simulink model "FPU_integrator"  (Simulink 7.6)
settings: Solver=FixedStepDiscrete  StartTime=0.0  StopTime=50  FixedStep=1  RelTol=1e-3
libraries: simulink x6
settings Model: Creator=jordan  LastModifiedBy=jordan
settings OptimizationCC: BlockReduction=off  ConditionallyExecuteInputs=off

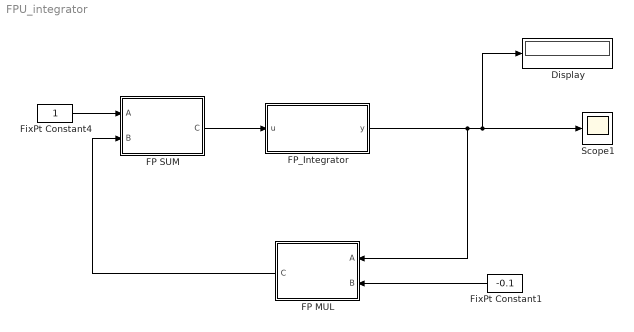
== system FPU_integrator ==
  Display : Display
  FP MUL : Subsystem
  FP SUM : Subsystem
  FP_Integrator : Subsystem
  FixPt Constant1 : Constant  DisableCoverage=on  Value=-0.1  OutDataTypeStr=single  LockScale=on
  FixPt Constant4 : Constant  DisableCoverage=on  OutDataTypeStr=single  LockScale=on
  Scope1 : Scope
      settings: SaveName=ScopeData3  MaxDataPoints=50000
  wires:
  FP_Integrator/1(y) -> Scope1/1, Display/1, FP MUL/1(A)
  FixPt Constant4/1 -> FP SUM/1(A)
  FixPt Constant1/1 -> FP MUL/2(B)
  FP SUM/1(C) -> FP_Integrator/1(u)
  FP MUL/1(C) -> FP SUM/2(B)

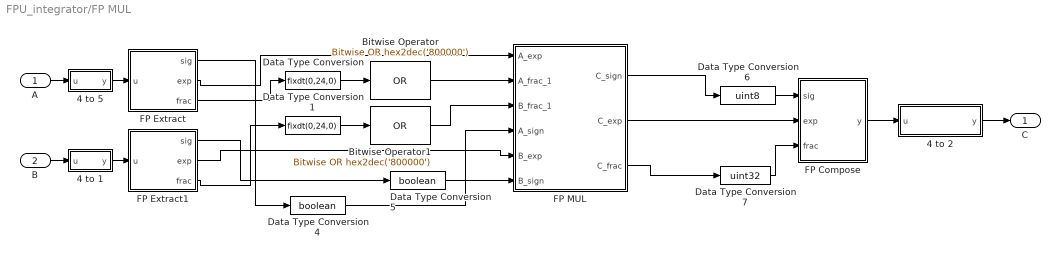
== system FPU_integrator/FP MUL ==
  A : Inport
  B : Inport  Port=2
  4 to 1 : Stateflow chart  TreatAsAtomicUnit=on
  4 to 2 : Stateflow chart  TreatAsAtomicUnit=on
  4 to 5 : Stateflow chart  TreatAsAtomicUnit=on
  Bitwise Operator : simulink/Logic and Bit Operations/Bitwise Operator  logicop=OR  UseBitMask=on  BitMask=hex2dec('800000')  BitMaskRealWorld=Stored Integer
  Bitwise Operator1 : simulink/Logic and Bit Operations/Bitwise Operator  logicop=OR  UseBitMask=on  BitMask=hex2dec('800000')  BitMaskRealWorld=Stored Integer
  Data Type Conversion : DataTypeConversion  OutDataTypeStr=fixdt(0,24,0)  RndMeth=Nearest
  Data Type Conversion1 : DataTypeConversion  OutDataTypeStr=fixdt(0,24,0)  RndMeth=Nearest
  Data Type Conversion4 : DataTypeConversion  OutDataTypeStr=boolean  RndMeth=Nearest
  Data Type Conversion5 : DataTypeConversion  OutDataTypeStr=boolean  RndMeth=Nearest
  Data Type Conversion6 : DataTypeConversion  OutDataTypeStr=uint8  RndMeth=Nearest
  Data Type Conversion7 : DataTypeConversion  OutDataTypeStr=uint32  RndMeth=Nearest
  FP Compose : Stateflow chart  TreatAsAtomicUnit=on
  FP Extract : Stateflow chart  TreatAsAtomicUnit=on
  FP Extract1 : Stateflow chart  TreatAsAtomicUnit=on
  FP MUL : Subsystem
  C : Outport  InitialOutput=0
  wires:
  Data Type Conversion7/1 -> FP Compose/3(frac)
  Data Type Conversion6/1 -> FP Compose/1(sig)
  FP Compose/1(y) -> 4 to 2/1(u)
  Data Type Conversion5/1 -> FP MUL/6(B_sign)
  Data Type Conversion4/1 -> FP MUL/4(A_sign)
  FP MUL/3(C_frac) -> Data Type Conversion7/1
  FP MUL/2(C_exp) -> FP Compose/2(exp)
  FP MUL/1(C_sign) -> Data Type Conversion6/1
  Bitwise Operator1/1 -> FP MUL/3(B_frac_1)
  Data Type Conversion1/1 -> Bitwise Operator1/1
  Bitwise Operator/1 -> FP MUL/2(A_frac_1)
  Data Type Conversion/1 -> Bitwise Operator/1
  FP Extract1/3(frac) -> Data Type Conversion1/1
  FP Extract/3(frac) -> Data Type Conversion/1
  FP Extract1/2(exp) -> FP MUL/5(B_exp)
  FP Extract/2(exp) -> FP MUL/1(A_exp)
  FP Extract1/1(sig) -> Data Type Conversion5/1
  FP Extract/1(sig) -> Data Type Conversion4/1
  B/1 -> 4 to 1/1(u)
  A/1 -> 4 to 5/1(u)
  4 to 5/1(y) -> FP Extract/1(u)
  4 to 1/1(y) -> FP Extract1/1(u)
  4 to 2/1(y) -> C/1

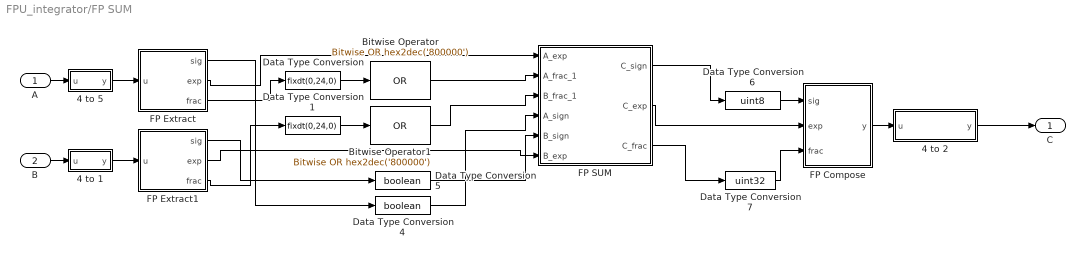
== system FPU_integrator/FP SUM ==
  A : Inport
  B : Inport  Port=2
  4 to 1 : Stateflow chart  TreatAsAtomicUnit=on
  4 to 2 : Stateflow chart  TreatAsAtomicUnit=on
  4 to 5 : Stateflow chart  TreatAsAtomicUnit=on
  Bitwise Operator : simulink/Logic and Bit Operations/Bitwise Operator  logicop=OR  UseBitMask=on  BitMask=hex2dec('800000')  BitMaskRealWorld=Stored Integer
  Bitwise Operator1 : simulink/Logic and Bit Operations/Bitwise Operator  logicop=OR  UseBitMask=on  BitMask=hex2dec('800000')  BitMaskRealWorld=Stored Integer
  Data Type Conversion : DataTypeConversion  OutDataTypeStr=fixdt(0,24,0)  RndMeth=Nearest
  Data Type Conversion1 : DataTypeConversion  OutDataTypeStr=fixdt(0,24,0)  RndMeth=Nearest
  Data Type Conversion4 : DataTypeConversion  OutDataTypeStr=boolean  RndMeth=Nearest
  Data Type Conversion5 : DataTypeConversion  OutDataTypeStr=boolean  RndMeth=Nearest
  Data Type Conversion6 : DataTypeConversion  OutDataTypeStr=uint8  RndMeth=Nearest
  Data Type Conversion7 : DataTypeConversion  OutDataTypeStr=uint32  RndMeth=Nearest
  FP Compose : Stateflow chart  TreatAsAtomicUnit=on
  FP Extract : Stateflow chart  TreatAsAtomicUnit=on
  FP Extract1 : Stateflow chart  TreatAsAtomicUnit=on
  FP SUM : Subsystem
  C : Outport  InitialOutput=0
  wires:
  A/1 -> 4 to 5/1(u)
  B/1 -> 4 to 1/1(u)
  FP Extract/1(sig) -> Data Type Conversion4/1
  FP Extract1/1(sig) -> Data Type Conversion5/1
  FP Extract/2(exp) -> FP SUM/1(A_exp)
  FP Extract1/2(exp) -> FP SUM/6(B_exp)
  FP Extract/3(frac) -> Data Type Conversion/1
  FP Extract1/3(frac) -> Data Type Conversion1/1
  Data Type Conversion/1 -> Bitwise Operator/1
  Bitwise Operator/1 -> FP SUM/2(A_frac_1)
  Data Type Conversion1/1 -> Bitwise Operator1/1
  Bitwise Operator1/1 -> FP SUM/3(B_frac_1)
  FP SUM/1(C_sign) -> Data Type Conversion6/1
  FP SUM/2(C_exp) -> FP Compose/2(exp)
  FP SUM/3(C_frac) -> Data Type Conversion7/1
  Data Type Conversion4/1 -> FP SUM/4(A_sign)
  Data Type Conversion5/1 -> FP SUM/5(B_sign)
  FP Compose/1(y) -> 4 to 2/1(u)
  Data Type Conversion6/1 -> FP Compose/1(sig)
  Data Type Conversion7/1 -> FP Compose/3(frac)
  4 to 5/1(y) -> FP Extract/1(u)
  4 to 1/1(y) -> FP Extract1/1(u)
  4 to 2/1(y) -> C/1

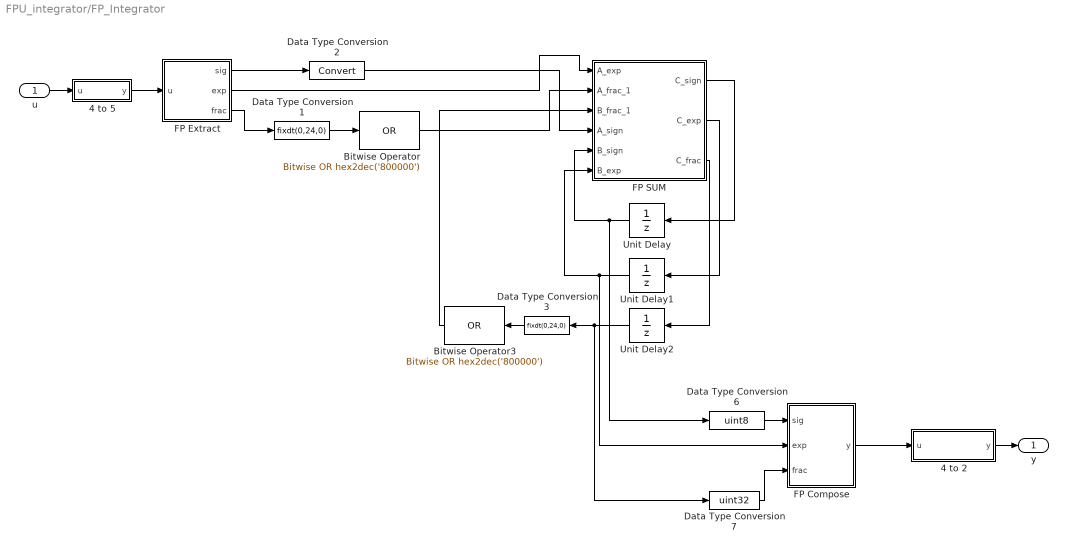
== system FPU_integrator/FP_Integrator ==
  u : Inport
  4 to 2 : Stateflow chart  TreatAsAtomicUnit=on
  4 to 5 : Stateflow chart  TreatAsAtomicUnit=on
  Bitwise Operator : simulink/Logic and Bit Operations/Bitwise Operator  logicop=OR  UseBitMask=on  BitMask=hex2dec('800000')  BitMaskRealWorld=Stored Integer
  Bitwise Operator3 : simulink/Logic and Bit Operations/Bitwise Operator  logicop=OR  UseBitMask=on  BitMask=hex2dec('800000')  BitMaskRealWorld=Stored Integer
  Data Type Conversion1 : DataTypeConversion  OutDataTypeStr=fixdt(0,24,0)  RndMeth=Nearest
  Data Type Conversion2 : DataTypeConversion  RndMeth=Nearest
  Data Type Conversion3 : DataTypeConversion  OutDataTypeStr=fixdt(0,24,0)  RndMeth=Nearest
  Data Type Conversion6 : DataTypeConversion  OutDataTypeStr=uint8  RndMeth=Nearest
  Data Type Conversion7 : DataTypeConversion  OutDataTypeStr=uint32  RndMeth=Nearest
  FP Compose : Stateflow chart  TreatAsAtomicUnit=on
  FP Extract : Stateflow chart  TreatAsAtomicUnit=on
  FP SUM : Subsystem
  Unit Delay : UnitDelay  SampleTime=-1
  Unit Delay1 : UnitDelay  SampleTime=-1
  Unit Delay2 : UnitDelay  SampleTime=-1
  y : Outport
  wires:
  FP SUM/1(C_sign) -> Unit Delay/1
  FP SUM/2(C_exp) -> Unit Delay1/1
  FP SUM/3(C_frac) -> Unit Delay2/1
  Unit Delay/1 -> FP SUM/5(B_sign), Data Type Conversion6/1
  Unit Delay1/1 -> FP SUM/6(B_exp), FP Compose/2(exp)
  Unit Delay2/1 -> Data Type Conversion3/1, Data Type Conversion7/1
  Data Type Conversion3/1 -> Bitwise Operator3/1
  Bitwise Operator3/1 -> FP SUM/3(B_frac_1)
  FP Extract/1(sig) -> Data Type Conversion2/1
  FP Extract/2(exp) -> FP SUM/1(A_exp)
  Data Type Conversion1/1 -> Bitwise Operator/1
  FP Extract/3(frac) -> Data Type Conversion1/1
  Bitwise Operator/1 -> FP SUM/2(A_frac_1)
  Data Type Conversion6/1 -> FP Compose/1(sig)
  Data Type Conversion7/1 -> FP Compose/3(frac)
  FP Compose/1(y) -> 4 to 2/1(u)
  4 to 5/1(y) -> FP Extract/1(u)
  Data Type Conversion2/1 -> FP SUM/4(A_sign)
  u/1 -> 4 to 5/1(u)
  4 to 2/1(y) -> y/1

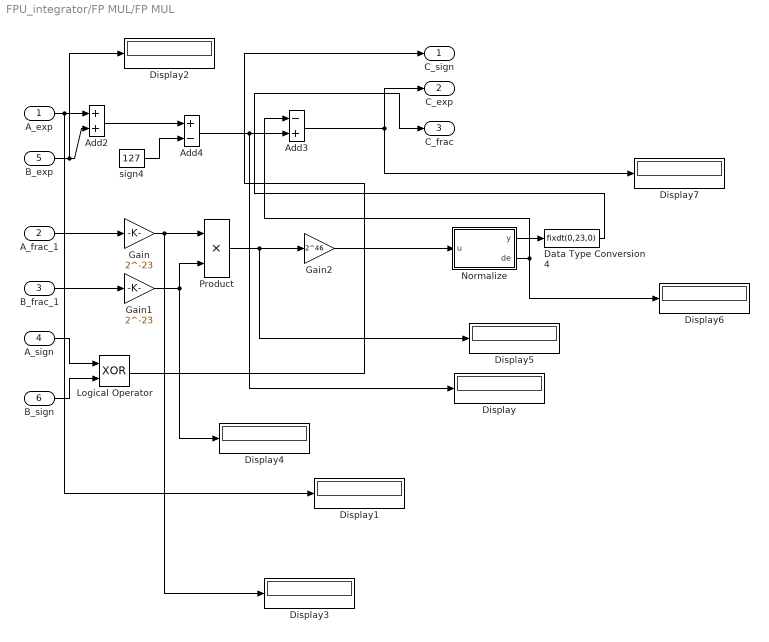
== system FPU_integrator/FP MUL/FP MUL ==
  A_exp : Inport  OutDataTypeStr=uint8
  A_frac_1 : Inport  Port=2  OutDataTypeStr=fixdt(0,24,0)
  B_frac_1 : Inport  Port=3  OutDataTypeStr=fixdt(0,24,0)
  A_sign : Inport  Port=4  OutDataTypeStr=boolean
  B_exp : Inport  Port=5  OutDataTypeStr=uint8
  B_sign : Inport  Port=6  OutDataTypeStr=boolean
  Add2 : Sum  OutDataTypeStr=fixdt(0,9,0)  RndMeth=Nearest
  Add3 : Sum  Inputs=-+  OutDataTypeStr=uint8  RndMeth=Nearest  SaturateOnIntegerOverflow=on
  Add4 : Sum  Inputs=+-  OutDataTypeStr=uint8  RndMeth=Nearest  SaturateOnIntegerOverflow=on
  Data Type Conversion4 : DataTypeConversion  OutDataTypeStr=fixdt(0,23,0)
  Display{,1..7} (8 alike) : Display
  Gain : Gain  Gain=2^-23  OutDataTypeStr=fixdt(0,24,23)  RndMeth=Nearest
  Gain1 : Gain  Gain=2^-23  OutDataTypeStr=fixdt(0,24,23)  RndMeth=Nearest
  Gain2 : Gain  Gain=2^46  OutDataTypeStr=fixdt(0,48,0)  RndMeth=Nearest
  Logical Operator : Logic  Operator=XOR  AllPortsSameDT=off  OutDataTypeStr=boolean
  Normalize : Stateflow chart  TreatAsAtomicUnit=on
  Product : Product  OutDataTypeStr=fixdt(0,48,46)  RndMeth=Nearest
  sign4 : Constant  Value=127  OutDataTypeStr=fixdt(0,9,0)
  C_sign : Outport  OutDataTypeStr=boolean
  C_exp : Outport  Port=2  OutDataTypeStr=uint8
  C_frac : Outport  Port=3  OutDataTypeStr=fixdt(0,23,0)
  wires:
  Gain2/1 -> Normalize/1(u)
  B_sign/1 -> Logical Operator/2
  A_exp/1 -> Display1/1, Add2/1
  A_sign/1 -> Logical Operator/1
  B_frac_1/1 -> Gain1/1
  A_frac_1/1 -> Gain/1
  Gain1/1 -> Display4/1, Product/2
  Gain/1 -> Display3/1, Product/1
  Add4/1 -> Display/1, Add3/2
  sign4/1 -> Add4/2
  Add2/1 -> Add4/1
  Product/1 -> Gain2/1, Display5/1
  Logical Operator/1 -> C_sign/1
  Data Type Conversion4/1 -> C_frac/1
  Add3/1 -> Display7/1, C_exp/1
  Normalize/2(de) -> Display6/1, Add3/1
  Normalize/1(y) -> Data Type Conversion4/1
  B_exp/1 -> Display2/1, Add2/2

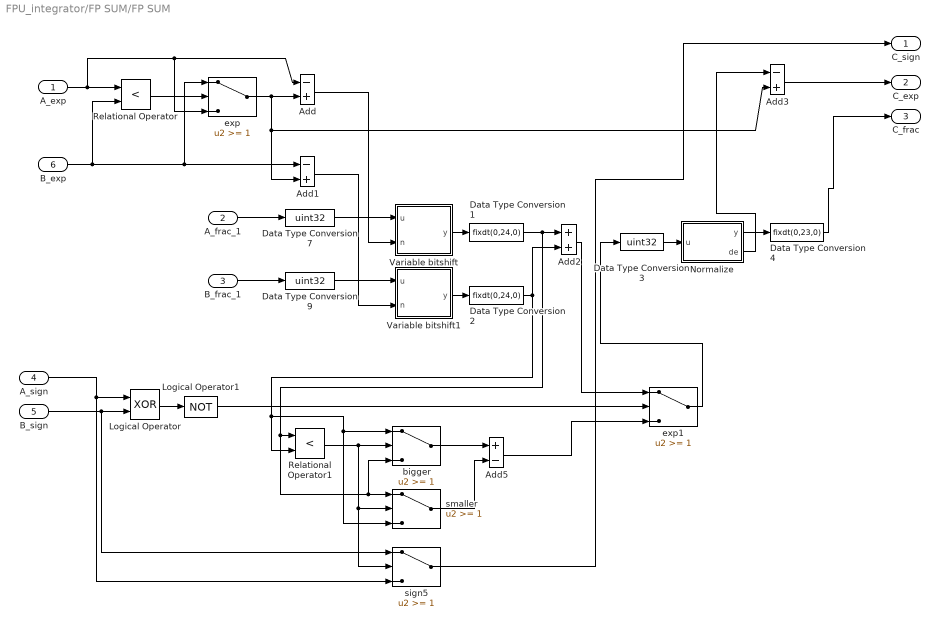
== system FPU_integrator/FP SUM/FP SUM ==
  A_exp : Inport  OutDataTypeStr=uint8
  A_frac_1 : Inport  Port=2  OutDataTypeStr=fixdt(0,24,0)
  B_frac_1 : Inport  Port=3  OutDataTypeStr=fixdt(0,24,0)
  A_sign : Inport  Port=4  OutDataTypeStr=boolean
  B_sign : Inport  Port=5  OutDataTypeStr=boolean
  B_exp : Inport  Port=6  OutDataTypeStr=uint8
  Add : Sum  Inputs=-+  OutDataTypeStr=int8
  Add1 : Sum  Inputs=-+  OutDataTypeStr=int8
  Add2 : Sum  OutDataTypeStr=fixdt(0,25,0)  RndMeth=Nearest
  Add3 : Sum  Inputs=-+  OutDataTypeStr=uint8  SaturateOnIntegerOverflow=on
  Add5 : Sum  Inputs=+-  OutDataTypeStr=fixdt(0,25,0)  RndMeth=Nearest
  Data Type Conversion1 : DataTypeConversion  OutDataTypeStr=fixdt(0,24,0)
  Data Type Conversion2 : DataTypeConversion  OutDataTypeStr=fixdt(0,24,0)
  Data Type Conversion3 : DataTypeConversion  OutDataTypeStr=uint32
  Data Type Conversion4 : DataTypeConversion  OutDataTypeStr=fixdt(0,23,0)
  Data Type Conversion7 : DataTypeConversion  OutDataTypeStr=uint32
  Data Type Conversion9 : DataTypeConversion  OutDataTypeStr=uint32
  Logical Operator : Logic  Operator=XOR  AllPortsSameDT=off  OutDataTypeStr=boolean
  Logical Operator1 : Logic  Operator=NOT  AllPortsSameDT=off  OutDataTypeStr=boolean
  Normalize : Stateflow chart  TreatAsAtomicUnit=on
  Relational Operator : RelationalOperator  Operator=<  OutDataTypeStr=boolean
  Relational Operator1 : RelationalOperator  Operator=<  OutDataTypeStr=boolean
  Variable bitshift : Stateflow chart  TreatAsAtomicUnit=on
  Variable bitshift1 : Stateflow chart  TreatAsAtomicUnit=on
  bigger : Switch  Threshold=1
  exp : Switch  Threshold=1
  exp1 : Switch  Threshold=1
  sign5 : Switch  Threshold=1
  smaller : Switch  Threshold=1
  C_sign : Outport  OutDataTypeStr=boolean
  C_exp : Outport  Port=2  OutDataTypeStr=uint8
  C_frac : Outport  Port=3  OutDataTypeStr=fixdt(0,23,0)
  wires:
  Add3/1 -> C_exp/1
  B_sign/1 -> sign5/1, Logical Operator/2
  A_sign/1 -> sign5/3, Logical Operator/1
  Data Type Conversion9/1 -> Variable bitshift1/1(u)
  Data Type Conversion7/1 -> Variable bitshift/1(u)
  sign5/1 -> C_sign/1
  exp1/1 -> Data Type Conversion3/1
  Add5/1 -> exp1/3
  smaller/1 -> Add5/2
  bigger/1 -> Add5/1
  Relational Operator1/1 -> sign5/2, smaller/2, bigger/2
  Logical Operator1/1 -> exp1/2
  Logical Operator/1 -> Logical Operator1/1
  Data Type Conversion4/1 -> C_frac/1
  Data Type Conversion3/1 -> Normalize/1(u)
  Normalize/2(de) -> Add3/1
  Normalize/1(y) -> Data Type Conversion4/1
  Add2/1 -> exp1/1
  Data Type Conversion2/1 -> smaller/3, bigger/1, Relational Operator1/2, Add2/2
  Variable bitshift1/1(y) -> Data Type Conversion2/1
  Add1/1 -> Variable bitshift1/2(n)
  Add/1 -> Variable bitshift/2(n)
  B_frac_1/1 -> Data Type Conversion9/1
  exp/1 -> Add3/2, Add1/2, Add/2
  Relational Operator/1 -> exp/2
  Data Type Conversion1/1 -> bigger/3, smaller/1, Relational Operator1/1, Add2/1
  Variable bitshift/1(y) -> Data Type Conversion1/1
  A_frac_1/1 -> Data Type Conversion7/1
  B_exp/1 -> Relational Operator/2, Add1/1, exp/1
  A_exp/1 -> Add/1, exp/3, Relational Operator/1

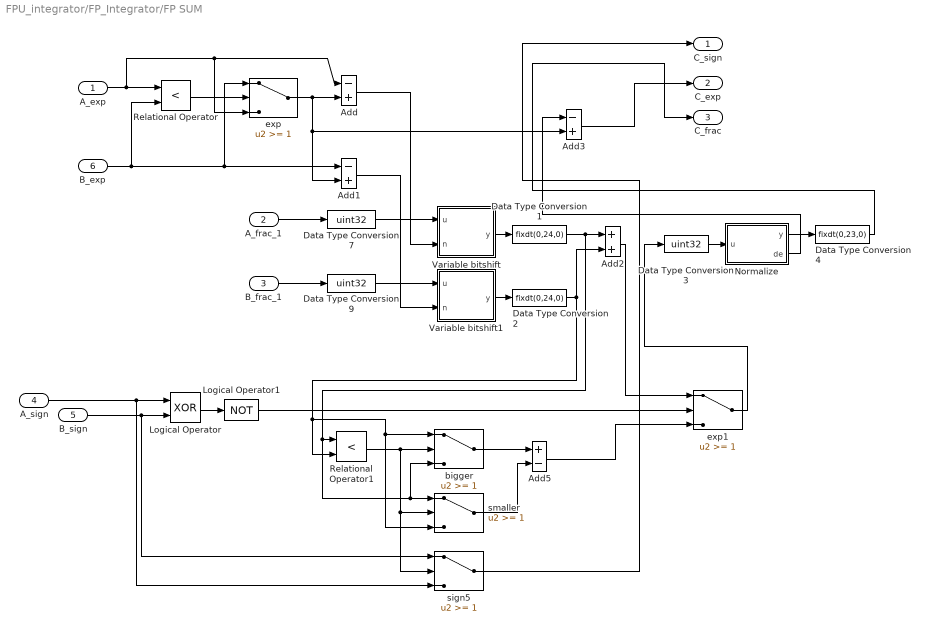
== system FPU_integrator/FP_Integrator/FP SUM ==
  A_exp : Inport  OutDataTypeStr=uint8
  A_frac_1 : Inport  Port=2  OutDataTypeStr=fixdt(0,24,0)
  B_frac_1 : Inport  Port=3  OutDataTypeStr=fixdt(0,24,0)
  A_sign : Inport  Port=4  OutDataTypeStr=boolean
  B_sign : Inport  Port=5  OutDataTypeStr=boolean
  B_exp : Inport  Port=6  OutDataTypeStr=uint8
  Add : Sum  Inputs=-+  OutDataTypeStr=int8
  Add1 : Sum  Inputs=-+  OutDataTypeStr=int8
  Add2 : Sum  OutDataTypeStr=fixdt(0,25,0)  RndMeth=Nearest
  Add3 : Sum  Inputs=-+  OutDataTypeStr=uint8  SaturateOnIntegerOverflow=on
  Add5 : Sum  Inputs=+-  OutDataTypeStr=fixdt(0,25,0)  RndMeth=Nearest
  Data Type Conversion1 : DataTypeConversion  OutDataTypeStr=fixdt(0,24,0)
  Data Type Conversion2 : DataTypeConversion  OutDataTypeStr=fixdt(0,24,0)
  Data Type Conversion3 : DataTypeConversion  OutDataTypeStr=uint32
  Data Type Conversion4 : DataTypeConversion  OutDataTypeStr=fixdt(0,23,0)
  Data Type Conversion7 : DataTypeConversion  OutDataTypeStr=uint32
  Data Type Conversion9 : DataTypeConversion  OutDataTypeStr=uint32
  Logical Operator : Logic  Operator=XOR  AllPortsSameDT=off  OutDataTypeStr=boolean
  Logical Operator1 : Logic  Operator=NOT  AllPortsSameDT=off  OutDataTypeStr=boolean
  Normalize : Stateflow chart  TreatAsAtomicUnit=on
  Relational Operator : RelationalOperator  Operator=<  OutDataTypeStr=boolean
  Relational Operator1 : RelationalOperator  Operator=<  OutDataTypeStr=boolean
  Variable bitshift : Stateflow chart  TreatAsAtomicUnit=on
  Variable bitshift1 : Stateflow chart  TreatAsAtomicUnit=on
  bigger : Switch  Threshold=1
  exp : Switch  Threshold=1
  exp1 : Switch  Threshold=1
  sign5 : Switch  Threshold=1
  smaller : Switch  Threshold=1
  C_sign : Outport  OutDataTypeStr=boolean
  C_exp : Outport  Port=2  OutDataTypeStr=uint8
  C_frac : Outport  Port=3  OutDataTypeStr=fixdt(0,23,0)
  wires:
  Add3/1 -> C_exp/1
  B_sign/1 -> sign5/1, Logical Operator/2
  A_sign/1 -> sign5/3, Logical Operator/1
  Data Type Conversion9/1 -> Variable bitshift1/1(u)
  Data Type Conversion7/1 -> Variable bitshift/1(u)
  sign5/1 -> C_sign/1
  exp1/1 -> Data Type Conversion3/1
  Add5/1 -> exp1/3
  smaller/1 -> Add5/2
  bigger/1 -> Add5/1
  Relational Operator1/1 -> sign5/2, smaller/2, bigger/2
  Logical Operator1/1 -> exp1/2
  Logical Operator/1 -> Logical Operator1/1
  Data Type Conversion4/1 -> C_frac/1
  Data Type Conversion3/1 -> Normalize/1(u)
  Normalize/2(de) -> Add3/1
  Normalize/1(y) -> Data Type Conversion4/1
  Add2/1 -> exp1/1
  Data Type Conversion2/1 -> smaller/3, bigger/1, Relational Operator1/2, Add2/2
  Variable bitshift1/1(y) -> Data Type Conversion2/1
  Add1/1 -> Variable bitshift1/2(n)
  Add/1 -> Variable bitshift/2(n)
  B_frac_1/1 -> Data Type Conversion9/1
  exp/1 -> Add3/2, Add1/2, Add/2
  Relational Operator/1 -> exp/2
  Data Type Conversion1/1 -> bigger/3, smaller/1, Relational Operator1/1, Add2/1
  Variable bitshift/1(y) -> Data Type Conversion1/1
  A_frac_1/1 -> Data Type Conversion7/1
  B_exp/1 -> Relational Operator/2, Add1/1, exp/1
  A_exp/1 -> Add/1, exp/3, Relational Operator/1

== matlab function FP_Integrator/FP SUM/Normalize ==
  data: u input uint32; y output uint32; de output double
function [y,de] = fcn(u)
%#eml

buf=u;
p=int8(-1);
c=bitand(buf,2^24);
for ind=1:25
    if (~c)
        p=p+1;
        buf=bitshift(buf,1);
        c=bitand(buf,2^24);
    end
end
bufy = bitand(bitshift(u,p),2^23-1);
y=bufy;
de=p;

== matlab function FP_Integrator/FP SUM/Variable bitshift ==
  data: u input uint32; y output uint32; n input int8
function y = fcn(u,n)
%#eml

y = bitshift(u,-n);

== matlab function FP SUM/FP Compose ==
  data: sig input uint8; exp input uint8; frac input uint32; y output uint32
function y = fcn(sig,exp,frac)
%#eml

z=uint32(0);
if sig
    z=uint32(bitshift(uint32(1),31));
end
buf=uint32(bitshift(uint32(exp),23));
z=bitor(z,buf);
z=bitor(z,frac);
y=z;

== matlab function FP SUM/FP Extract ==
  data: u input uint32; sig output uint8; exp output uint8; frac output uint32
function [sig,exp,frac] = fcn(u)
%#eml

z=u;
sig=uint8(bitshift(z,-31));
exp=uint8(bitshift(bitshift(z,1),-24));
frac=uint32(bitand(z,8388607));
%bexp=uint8(bitshift(bitshift(z,1),-23));
% exp1=uint8(zeros(8,1));
% frac1=uint8(zeros(23,1));
% for ind=0:7
%     exp1(ind+1)=uint8(bitand(bitshift(bexp,-ind),1));
% end
% bfrac=z;
% for ind=0:22
%     frac1(ind+1)=uint8(bitand(bitshift(bfrac,-ind),1));
% end
% exp=exp1;
% frac=frac1;

== matlab function FP SUM/FP Extract1 ==
  data: u input uint32; sig output uint8; exp output uint8; frac output uint32
function [sig,exp,frac] = fcn(u)
%#eml

z=u;
sig=uint8(bitshift(z,-31));
exp=uint8(bitshift(bitshift(z,1),-24));
frac=uint32(bitand(z,8388607));
%bexp=uint8(bitshift(bitshift(z,1),-23));
% exp1=uint8(zeros(8,1));
% frac1=uint8(zeros(23,1));
% for ind=0:7
%     exp1(ind+1)=uint8(bitand(bitshift(bexp,-ind),1));
% end
% bfrac=z;
% for ind=0:22
%     frac1(ind+1)=uint8(bitand(bitshift(bfrac,-ind),1));
% end
% exp=exp1;
% frac=frac1;

== matlab function FP_Integrator/FP SUM/Variable bitshift1 ==
  data: u input uint32; y output uint32; n input int8
function y = fcn(u,n)
%#eml

y = bitshift(u,-n);

== matlab function FP SUM/FP SUM/Normalize ==
  data: u input uint32; y output uint32; de output double
function [y,de] = fcn(u)
%#eml

buf=u;
p=int8(-1);
c=bitand(buf,2^24);
for ind=1:25
    if (~c)
        p=p+1;
        buf=bitshift(buf,1);
        c=bitand(buf,2^24);
    end
end
bufy = bitand(bitshift(u,p),2^23-1);
y=bufy;
de=p;

== matlab function FP_Integrator/FP Extract ==
  data: u input uint32; sig output uint8; exp output uint8; frac output uint32
function [sig,exp,frac] = fcn(u)
%#eml

z=u;
sig=uint8(bitshift(z,-31));
exp=uint8(bitshift(bitshift(z,1),-24));
frac=uint32(bitand(z,8388607));
%bexp=uint8(bitshift(bitshift(z,1),-23));
% exp1=uint8(zeros(8,1));
% frac1=uint8(zeros(23,1));
% for ind=0:7
%     exp1(ind+1)=uint8(bitand(bitshift(bexp,-ind),1));
% end
% bfrac=z;
% for ind=0:22
%     frac1(ind+1)=uint8(bitand(bitshift(bfrac,-ind),1));
% end
% exp=exp1;
% frac=frac1;

== matlab function FP MUL/FP MUL/Normalize ==
  data: u input fixdt(0,48,0); y output uint32; de output double
function [y,de] = fcn(u)
%#eml

buf=u;
p=int8(-1);
c=bitand(buf,fi(2^47,0,48,0));
for ind=1:25
    if (c==0)
        p=p+1;
        buf=bitshift(buf,1);
        c=bitand(buf,fi(2^47,0,48,0));
    end
end
bufy = bitand(bitshift(u,p),fi(2^46-1,0,48,0));
y=uint32(bitshift(bufy,-23));
de=p;

== matlab function FP_Integrator/FP Compose ==
  data: sig input uint8; exp input uint8; frac input uint32; y output uint32
function y = fcn(sig,exp,frac)
%#eml

z=uint32(0);
if sig
    z=uint32(bitshift(uint32(1),31));
end
buf=uint32(bitshift(uint32(exp),23));
z=bitor(z,buf);
z=bitor(z,frac);
y=z;

== matlab function FP MUL/FP Extract ==
  data: u input uint32; sig output uint8; exp output uint8; frac output uint32
function [sig,exp,frac] = fcn(u)
%#eml

z=u;
sig=uint8(bitshift(z,-31));
exp=uint8(bitshift(bitshift(z,1),-24));
frac=uint32(bitand(z,8388607));
%bexp=uint8(bitshift(bitshift(z,1),-23));
% exp1=uint8(zeros(8,1));
% frac1=uint8(zeros(23,1));
% for ind=0:7
%     exp1(ind+1)=uint8(bitand(bitshift(bexp,-ind),1));
% end
% bfrac=z;
% for ind=0:22
%     frac1(ind+1)=uint8(bitand(bitshift(bfrac,-ind),1));
% end
% exp=exp1;
% frac=frac1;

== matlab function FP MUL/FP Extract1 ==
  data: u input uint32; sig output uint8; exp output uint8; frac output uint32
function [sig,exp,frac] = fcn(u)
%#eml

z=u;
sig=uint8(bitshift(z,-31));
exp=uint8(bitshift(bitshift(z,1),-24));
frac=uint32(bitand(z,8388607));
%bexp=uint8(bitshift(bitshift(z,1),-23));
% exp1=uint8(zeros(8,1));
% frac1=uint8(zeros(23,1));
% for ind=0:7
%     exp1(ind+1)=uint8(bitand(bitshift(bexp,-ind),1));
% end
% bfrac=z;
% for ind=0:22
%     frac1(ind+1)=uint8(bitand(bitshift(bfrac,-ind),1));
% end
% exp=exp1;
% frac=frac1;

== matlab function FP SUM/FP SUM/Variable bitshift ==
  data: u input uint32; y output uint32; n input int8
function y = fcn(u,n)
%#eml

y = bitshift(u,-n);

== matlab function FP MUL/FP Compose ==
  data: sig input uint8; exp input uint8; frac input uint32; y output uint32
function y = fcn(sig,exp,frac)
%#eml

z=uint32(0);
if sig
    z=uint32(bitshift(uint32(1),31));
end
buf=uint32(bitshift(uint32(exp),23));
z=bitor(z,buf);
z=bitor(z,frac);
y=z;

== matlab function FP_Integrator/4 to 2 ==
  data: y output single; u input uint32
function y  = fcn(u)
%#eml
y=typecast(u,'single');

== matlab function FP SUM/FP SUM/Variable bitshift1 ==
  data: u input uint32; y output uint32; n input int8
function y = fcn(u,n)
%#eml

y = bitshift(u,-n);

== matlab function FP SUM/4 to 5 ==
  data: y output uint32; u input single
function y  = fcn(u)
%#eml
y=typecast(u,'uint32');

== matlab function FP_Integrator/4 to 5 ==
  data: y output uint32; u input single
function y  = fcn(u)
%#eml
y=typecast(u,'uint32');

== matlab function FP SUM/4 to 1 ==
  data: y output uint32; u input single
function y  = fcn(u)
%#eml
y=typecast(u,'uint32');

== matlab function FP MUL/4 to 5 ==
  data: y output uint32; u input single
function y  = fcn(u)
%#eml
y=typecast(u,'uint32');

== matlab function FP MUL/4 to 1 ==
  data: y output uint32; u input single
function y  = fcn(u)
%#eml
y=typecast(u,'uint32');

== matlab function FP SUM/4 to 2 ==
  data: y output single; u input uint32
function y  = fcn(u)
%#eml
y=typecast(u,'single');

== matlab function FP MUL/4 to 2 ==
  data: y output single; u input uint32
function y  = fcn(u)
%#eml
y=typecast(u,'single');
